simulink library "PouchCellAMP20M1HD"  (R2024a)
settings: Solver=VariableStepAuto  StartTime=0.0  StopTime=10.0  RelTol=1e-3
libraries: fl_lib x6, batteryecm_lib x1
settings Model: Creator=Carlos  LastModifiedBy=Carlos

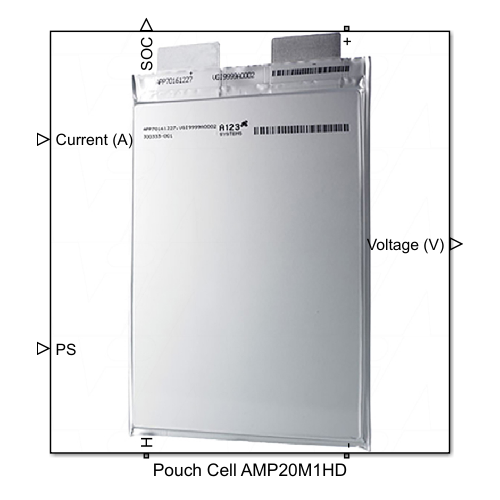
[thumbnail: Simulink's stored preview of the top-level diagram]
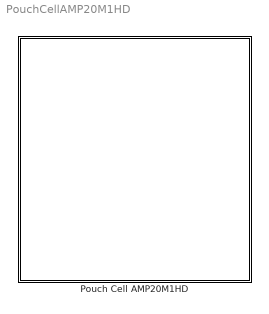
== system PouchCellAMP20M1HD ==
  Pouch Cell AMP20M1HD : Subsystem
      settings: PortSchema="{\"entries\":[{\"content\":{\"sides\":[{\"content\":{\"connectorIds\":[\"LConn1\",\"LConn2\"]},\"type\":\"ConnectorPlacement.EquallySpacedRectSide\",\"uuid\":\"1ad4bd77-f3cd-4a33-b1f1-8549cde45efa\"},{\"content\":{\"connectorIds\":[\"RConn1\"],\"side\":\"RIGHT\"},\"type\":\"ConnectorPlacement.EquallySpacedRectSide\",\"uuid\":\"9571ac2f-f2ec-4c0a-999c-8ea72e2cf4ad\"},{\"content\":{\"connectorIds\":[\"LConn3\",\"LConn4\"],\"side\":\"TOP\"},\"type\":\"ConnectorPlacement.EquallySpacedRectSide\",\"uuid\":\"d345a9ac-e4a8-4cf5-b4f6-097232c3cb5c\"},{\"content\":{\"connectorIds\":[\"RConn2\",\"RConn3\"],\"side\":\"BOTTOM\"},\"type\":\"ConnectorPlacement.EquallySpacedRectSide\",\"uuid\":\"7baf50c1-841c-4e4e-b39d-add364b405c0\"}]},\"type\":\"ConnectorPlacement.EquallySpacedConnector\",\"uuid\":\"1a2d2ccb-b2c1-437b-8298-ee46cad3b357\"}],\"packageUris\":[\"http://schema.mathworks.com/mf0/Connector/R2020b\"],\"version\":\"1.0\"}"
      mask Display: image('AMP20M1HD.jpg');

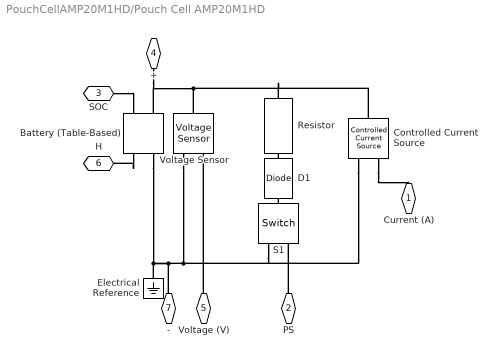
== system PouchCellAMP20M1HD/Pouch Cell AMP20M1HD ==
  Battery (Table-Based) : batteryecm_lib/Battery (Table-Based)  Tag={'toolbox/physmod/battery/shared_library/m/batteryecm_lib_parts';'Battery__Table_Based_/A123/AMP20M1HD.xml'}  SOC_vec=SOC_vec  T_dependence=simscape.enum.tablebattery.temperature_dependence.yes  prm_dir=simscape.enum.tablebattery.prm_dir.noCurrentDirectionality  T_vec=T_vec K  V0_mat=V0_mat V  V0_vec=[2.93217 2.94263 2.95309 2.96355 2.97401 2.98447 2.99493 3.02455 3.05382 3.07377 3.08453 3.09529 3.09916 3.10271 3.10625 3.1098 3.11335 3.11689 3.12044 3.13089 3.13795 3.14459 3.14961 3.15451 3.15932 3.16324 3.16716 3.17063 3.17297 3.17544 3.17798 3.18052 3.18295 3.18533 3.18771 3.19009 3.19215 3.19403 3.1959 3.19777 3.1998 3.20198 3.20371 3.20501 3.20619 3.20738 3.20856 3.20974 3.21092 3.2121 3.21329 3.21447 3.21565 3.21672 3.21787 3.21904 3.22021 3.22139 3.22256 3.22374 3.22492 3.2261 3.22728 3.22847 3.22965 3.23083 3.23201 3.23319 3.23437 3.23552 3.23652 3.23778 3.23909 3.24045 3.24217 3.2439 3.24563 3.24736 3.24909 3.25082 3.25255 3.25428 3.256 3.25774 3.25951 3.26116 3.26238 3.26307 3.26352 3.26396 3.26441 3.26485 3.2653 3.26593 3.26612 3.26743 3.26879 3.27596 3.2842 3.30299 3.33677] V  V_range=[1.8 Inf] V  R0_mat=R0_mat Ohm  R0_vec=[0.00349 0.0033 0.00311 0.00292 0.00272 0.00253 0.00235 0.00233 0.00235 0.00232 0.00223 0.00214 0.00205 0.00196 0.00187 0.00181 0.00175 0.00169 0.00164 0.00167 0.00168 0.00168 0.00168 0.00168 0.00167 0.00167 0.00167 0.00167 0.00166 0.00165 0.00164 0.00164 0.00163 0.00163 0.00162 0.00162 0.00161 0.0016 0.00159 0.00159 0.00158 0.00158 0.00158 0.00157 0.00156 0.00156 0.00155 0.00154 0.00154 0.00153 0.00153 0.00152 0.00151 0.00151 0.0015 0.0015 0.0015 0.00149 0.00149 0.00149 0.00148 0.00148 0.00148 0.00147 0.00147 0.00147 0.00147 0.00146 0.00146 0.00146 0.00145 0.00146 0.00146 0.00147 0.00147 0.00148 0.00149 0.0015 0.0015 0.00151 0.00152 0.00153 0.00153 0.00154 0.00155 0.00155 0.00156 0.00155 0.00154 0.00153 0.00152 0.00151 0.0015 0.00148 0.00144 0.0014 0.00137 0.00136 0.00131 0.00127 0.00104] Ohm  R0_dis_mat=[.0117, .0085, .009; .011, .0085, .009; .0114, .0087, .0092; .0107, .0082, .0088; .0107, .0083, .0091; .0113, .0085, .0089; .0116, .0085, .0089] % Parameter not set Ohm  R0_dis_vec=[.0085, .0085, .0087, .0082, .0083, .0085, .0085] % Parameter not set Ohm  R0_ch_mat=[.0117, .0085, .009; .011, .0085, .009; .0114, .0087, .0092; .0107, .0082, .0088; .0107, .0083, .0091; .0113, .0085, .0089; .0116, .0085, .0089] % Parameter not set Ohm  R0_ch_vec=[.0085, .0085, .0087, .0082, .0083, .0085, .0085] % Parameter not set Ohm  AH=AH hr*A  prm_leak=simscape.enum.tablebattery.prm_leak.disabled  Rleak_vec=[8000, 7000, 6000] % Parameter not set Ohm  Rleak=7e3 % Parameter not set Ohm  extrapolation_option=simscape.enum.extrapolation.nearest  SOC_port=simscape.enum.tablebattery.enable.yes  prm_dyn=simscape.enum.tablebattery.prm_dyn.rc1  R1_mat=R1_mat Ohm  R1_vec=[.0029, .0024, .0026, .0016, .0023, .0018, .0017] % Parameter not set Ohm  tau1_mat=tau1_mat s  tau1_vec=[36, 45, 105, 29, 77, 33, 39] % Parameter not set s  R2_mat=[.0109, .0029, .0013; .0069, .0024, .0012; .0047, .0026, .0013; .0034, .0016, .001; .0033, .0023, .0014; .0033, .0018, .0011; .0028, .0017, .0011] % Parameter not set Ohm  R2_vec=[.0029, .0024, .0026, .0016, .0023, .0018, .0017] % Parameter not set Ohm  tau2_mat=[20, 36, 39; 31, 45, 39; 109, 105, 61; 36, 29, 26; 59, 77, 67; 40, 33, 29; 25, 39, 33] % Parameter not set s  tau2_vec=[36, 45, 105, 29, 77, 33, 39] % Parameter not set s  R3_mat=[.0109, .0029, .0013; .0069, .0024, .0012; .0047, .0026, .0013; .0034, .0016, .001; .0033, .0023, .0014; .0033, .0018, .0011; .0028, .0017, .0011] % Parameter not set Ohm  R3_vec=[.0029, .0024, .0026, .0016, .0023, .0018, .0017] % Parameter not set Ohm  tau3_mat=[20, 36, 39; 31, 45, 39; 109, 105, 61; 36, 29, 26; 59, 77, 67; 40, 33, 29; 25, 39, 33] % Parameter not set s  tau3_vec=[36, 45, 105, 29, 77, 33, 39] % Parameter not set s  R4_mat=[.0109, .0029, .0013; .0069, .0024, .0012; .0047, .0026, .0013; .0034, .0016, .001; .0033, .0023, .0014; .0033, .0018, .0011; .0028, .0017, .0011] % Parameter not set Ohm  R4_vec=[.0029, .0024, .0026, .0016, .0023, .0018, .0017] % Parameter not set Ohm  tau4_mat=[20, 36, 39; 31, 45, 39; 109, 105, 61; 36, 29, 26; 59, 77, 67; 40, 33, 29; 25, 39, 33] % Parameter not set s  tau4_vec=[36, 45, 105, 29, 77, 33, 39] % Parameter not set s  R5_mat=[.0109, .0029, .0013; .0069, .0024, .0012; .0047, .0026, .0013; .0034, .0016, .001; .0033, .0023, .0014; .0033, .0018, .0011; .0028, .0017, .0011] % Parameter not set Ohm  R5_vec=[.0029, .0024, .0026, .0016, .0023, .0018, .0017] % Parameter not set Ohm  tau5_mat=[20, 36, 39; 31, 45, 39; 109, 105, 61; 36, 29, 26; 59, 77, 67; 40, 33, 29; 25, 39, 33] % Parameter not set s  tau5_vec=[36, 45, 105, 29, 77, 33, 39] % Parameter not set s  prm_fade=simscape.enum.tablebattery.prm_fade.tableNandT  N0=100 % Parameter not set  dV0=0 % Parameter not set  dR0=0 % Parameter not set  dAH=0 % Parameter not set  dRleak=0 % Parameter not set  dR1=0 % Parameter not set  dR2=0 % Parameter not set  dR3=0 % Parameter not set  dR4=0 % Parameter not set  dR5=0 % Parameter not set  N0vec=N0vec  Tfadevec=Tfadevec K  dV0vec=[0 -0.3227 -0.6453 -0.9509 -1.1187 -1.2594 -1.4 -1.5407 -1.6219 -1.683 -1.7439 -1.8049 -1.8602 -1.9134 -1.9665 -2.0196 -2.0441 -2.0544 -2.0647 -2.075 -2.085 -2.0949 -2.1048 -2.1146 -2.1183 -2.1198 -2.1212 -2.1226 -2.1259 -2.1303 -2.1347 -2.1391 -2.1431 -2.1462 -2.1493 -2.1524 -2.1556 -2.1591 -2.1625 -2.166 -2.1695 -2.1729 -2.1764 -2.1798 -2.1833 -2.1867 -2.1902 -2.1936 -2.197 -2.2002 -2.2034 -2.2067 -2.2106 -2.2156 -2.2206 -2.2256 -2.2316 -2.2405 -2.2493 -2.2582 -2.2676 -2.2798 -2.292 -2.3042 -2.3164 -2.3294 -2.3424 -2.3556 -2.3688 -2.3818 -2.3947 -2.4077 -2.4207 -2.4336 -2.4465 -2.4594 -2.4722 -2.485 -2.4978 -2.5106 -2.5233 -2.5361 -2.5489 -2.5617 -2.5745 -2.5872 -2.5999 -2.6126 -2.6253 -2.6381 -2.6508 -2.6635 -2.6765 -2.6898 -2.703 -2.7163 -2.7295 -2.7428 -2.756 -2.7693]  dR0vec=[0 0 0 0 0 0 0 0 0 0 0 0 0 0 0 0 0 0 0 0 0 0 0 0 0 0 0 0 0 0 0 0 0 0 0 0 0 0 0 0 0 0 0 0 0 0 0 0 0 0 0 0 0 0 0 0 0 0 0 0 0 0 0 0 0 0 0 0 0 0 0 0 0 0 0 0 0 0 0 0 0 0 0 0 0 0 0 0 0 0 0 0 0 0 0 0 0 0 0 0] % Parameter assumed  dAHvec=[0 -0.319 -0.638 -0.939 -1.189 -1.439 -1.688 -1.938 -2.188 -2.435 -2.682 -2.93 -3.177 -3.424 -3.671 -3.918 -4.169 -4.421 -4.673 -4.925 -5.177 -5.429 -5.681 -5.933 -6.185 -6.437 -6.683 -6.917 -7.152 -7.386 -7.621 -7.855 -8.09 -8.324 -8.558 -8.793 -9.033 -9.292 -9.551 -9.809 -10.068 -10.327 -10.586 -10.845 -11.104 -11.363 -11.622 -11.88 -12.132 -12.374 -12.616 -12.857 -13.099 -13.341 -13.582 -13.824 -14.066 -14.307 -14.549 -14.791 -15.035 -15.281 -15.526 -15.772 -16.017 -16.263 -16.508 -16.757 -17.007 -17.256 -17.506 -17.755 -18.005 -18.254 -18.504 -18.752 -18.999 -19.246 -19.493 -19.74 -19.986 -20.233 -20.48 -20.727 -20.973 -21.219 -21.464 -21.71 -21.955 -22.201 -22.446 -22.692 -22.943 -23.199 -23.455 -23.711 -23.966 -24.222 -24.478 -24.733]  dRleakvec=[0, 0, 0, 0] % Parameter not set  dR1vec=[0, 0, 0, 0] % Parameter not set  dR2vec=[0, 0, 0, 0] % Parameter not set  dR3vec=[0, 0, 0, 0] % Parameter not set  dR4vec=[0, 0, 0, 0] % Parameter not set  dR5vec=[0, 0, 0, 0] % Parameter not set  dV0mat=dV0mat  dR0mat=dR0mat  dAHmat=dAHmat  dRleakmat=[0, 0; 0, 0; 0, 0; 0, 0] % Parameter not set  dR1mat=dR1mat  dR2mat=[0, 0; 0, 0; 0, 0; 0, 0] % Parameter not set  dR3mat=[0, 0; 0, 0; 0, 0; 0, 0] % Parameter not set  dR4mat=[0, 0; 0, 0; 0, 0; 0, 0] % Parameter not set  dR5mat=[0, 0; 0, 0; 0, 0; 0, 0] % Parameter not set  prm_age_modeling=simscape.enum.tablebattery.prm_age_modeling.tableTandTime  storage_dt_age_vec=storage_dt_age_vec d  storage_T_age_vec=storage_T_age_vec K  prm_age_OCV=simscape.enum.tablebattery.prm_age_OCV.OCV  OCV_age=0.9 % Parameter not set  SOC_age=0.6 % Parameter not set  prm_age_resistance=simscape.enum.tablebattery.prm_age.disabled  OCV_scaling_age_resistance=2.2134e6 % Parameter not set  OCV_offset_age_resistance=1.632e6 % Parameter not set  temp_exp_age_resistance=0.515833569 % Parameter not set V  t_exp_age_resistance=0.75 % Parameter not set  T_age_vec_resistance=[273.15, 298.15, 323.15] % Parameter not set K  dt_age_vec_resistance=[0, 90, 180, 270] % Parameter not set d  dR0_age_vec=[0, 0, 0] % Parameter not set  t_meas_dR0_age=100 % Parameter not set d  dR0_age_mat=[0, 0, 0; 0, 0, 0; 0, 0, 0; 0, 0, 0] % Parameter not set  prm_age_capacity=simscape.enum.tablebattery.prm_age.enabled  OCV_scaling_age_capacity=1.5097e07 % Parameter not set  OCV_offset_age_capacity=8.3625e06 % Parameter not set  temp_exp_age_capacity=0.6011 % Parameter not set V  t_exp_age_capacity=0.75 % Parameter not set  T_age_vec_capacity=T_age_vec_capacity K  dt_age_vec_capacity=dt_age_vec_capacity d  dAH_age_vec=[0, 0, 0] % Parameter not set  t_meas_dAH_age=100 % Parameter not set d  dAH_age_mat=dAH_age_mat  thermal_port=simscape.enum.thermaleffects.model  temperature=298.15 % Parameter not set K  thermal_mass=446.4 % Parameter assumed J/K  i_specify=on  i_priority=None  i=i A  i_nominal_specify=off  i_nominal_value=1  i_nominal_unit=A  v_specify=on  v_priority=None  v=v V  v_nominal_specify=on  v_nominal_value=v_nominal_value  v_nominal_unit=V  stateOfCharge_specify=on  stateOfCharge_priority=High  stateOfCharge=initialSOC  stateOfCharge_nominal_specify=on  stateOfCharge_nominal_value=finalSOC  stateOfCharge_nominal_unit=1  num_cycles_specify=on  num_cycles_priority=High  num_cycles=num_cycles  num_cycles_nominal_specify=on  num_cycles_nominal_value=num_cycles_nominal_value  num_cycles_nominal_unit=1  cell_temperature_specify=on  cell_temperature_priority=High  cell_temperature=cell_temperature K  cell_temperature_nominal_specify=off  cell_temperature_nominal_value=1  cell_temperature_nominal_unit=K
      settings: AttributesFormatString=A123:AMP20M1HD
  Controlled Current Source : fl_lib/Electrical/Electrical Sources/Controlled Current Source
  D1 : fl_lib/Electrical/Electrical Elements/Diode  Vf=0.6 V  Ron=0.3 Ohm  Goff=1e-8 1/Ohm  i_specify=off  i_priority=None  i=0 A  i_nominal_specify=off  i_nominal_value=1  i_nominal_unit=A  v_specify=off  v_priority=None  v=0 V  v_nominal_specify=off  v_nominal_value=1  v_nominal_unit=V
      settings: LogSimulationData=on
  Electrical Reference : fl_lib/Electrical/Electrical Elements/Electrical Reference
  Resistor : fl_lib/Electrical/Electrical Elements/Resistor  R=10 Ohm  i_specify=off  i_priority=None  i=0 A  i_nominal_specify=off  i_nominal_value=1  i_nominal_unit=A  v_specify=off  v_priority=None  v=0 V  v_nominal_specify=off  v_nominal_value=1  v_nominal_unit=V
  S1 : fl_lib/Electrical/Electrical Elements/Switch  R_closed=0.01 Ohm  G_open=1e-8 1/Ohm  Threshold=0.5  i_specify=off  i_priority=None  i=0 A  i_nominal_specify=off  i_nominal_value=1  i_nominal_unit=A  v_specify=off  v_priority=None  v=0 V  v_nominal_specify=off  v_nominal_value=1  v_nominal_unit=V
  Voltage Sensor : fl_lib/Electrical/Electrical Sensors/Voltage Sensor
  Current (A) : PMIOPort  Side=Left
  PS : PMIOPort  Port=2  Side=Left
  SOC : PMIOPort  Port=3  Side=Left
  + : PMIOPort  Port=4  Side=Left
  Voltage (V) : PMIOPort  Port=5  Side=Right
  H : PMIOPort  Port=6  Side=Right
  - : PMIOPort  Port=7  Side=Right
  connections:
  SOC/RConn1 -- Battery (Table-Based)/LConn2
  Voltage Sensor/LConn1 -- Battery (Table-Based)/LConn1 -- +/RConn1 -- Resistor/LConn1 -- Controlled Current Source/LConn1
  Electrical Reference/LConn1 -- Controlled Current Source/RConn2 -- S1/RConn2 -- Voltage Sensor/RConn2 -- -/RConn1 -- Battery (Table-Based)/RConn1
  Battery (Table-Based)/RConn2 -- H/RConn1
  Voltage (V)/RConn1 -- Voltage Sensor/RConn1
  Controlled Current Source/RConn1 -- Current (A)/RConn1
  S1/LConn1 -- D1/RConn1
  PS/RConn1 -- S1/RConn1
  D1/LConn1 -- Resistor/RConn1
